simulink model "Australian14gen_inertia"  (R2017b)
settings: Solver=ode23tb  StartTime=0.0  StopTime=50  FixedStep=1e-3  RelTol=1e-3  AbsTol=1e-3  EnableMultiTasking=on
PreLoadFcn:
  | dataaustralian14gen
values from neighbouring files (symbols this model uses):
  alpha = -sys.follin.opt.alpha*1e8    [main_following.m]    (also in optimgains.mat = [-2447350365.29 -12566370614.4 -12566370614.4 -11730281347.7)
  bus_v = [ 101	15 ... (first row only)    [dataaustralian14gen.m]
  comp = [ 1	211	0	0 ... (first row only)    [dataaustralian14gen.m]
  dist = sys.follin.dist    [main_following.m]    (also in main_forming.m = sys.formin.dist)
  Exc = [ 101	0	 200	0.1	    13.25  2.5	 0	0       0       0       0       0 ... (first row only)    [dataaustralian14gen.m]
  FH = 13    [dataaustralian14gen.m]
  FI = 1    [dataaustralian14gen.m]
  FL = .1    (= 0.1)    [dataaustralian14gen.m]
  G_data = [ 101	333.3	15	3.6	0.14	1.1	0.65	0.25	8.5     0.25	0.05	0       0       0.25	0.2 	0 ... (first row only)    [dataaustralian14gen.m]
  KH = 120    [dataaustralian14gen.m]
  KI = 10    [dataaustralian14gen.m]
  KL = 10    [dataaustralian14gen.m]
  Kvsc = [-4.89904313526 -21.043852985 -7.4754770322 -20.8245159401 -7.65455531538 -20.65157337 -7.20128124012 -20.8334958357 -6.74777960012 -20.6206111903 -7.78863485578 -20.7555924998 ... (30 elements, 2x15)]    [optimgains.mat]
  line = [ 102	217	0.0084	0.0667	0.817	330	1 ... (first row only)    [dataaustralian14gen.m]
  load_mag = load_case4    [dataaustralian14gen.m]
  p = p_case4    [dataaustralian14gen.m]
  Pinit = zeros(15,1)    [dataaustralian14gen.m]
  PLL_Ki = 2/500    (= 0.004)    [dataaustralian14gen.m]
  PLL_Kp = 2/500    (= 0.004)    [dataaustralian14gen.m]
  PSSMODEL = 1    [dataaustralian14gen.m]
  trans = [ 1	101	102	15	330	333.3	12	12 ... (first row only)    [dataaustralian14gen.m]
undefined symbols (not defined in the file or in its folder): D1, Delta, sys, thetavsc0, Vbase
libraries: powerlib x388, Library x60, powerlib_meascontrol x15, sps_avr x10, powerlib_extras x4
(part 5 of 5)

== system Australian14gen_inertia/VI504_form ==
  Complex to Magnitude-Angle : ComplexToMagnitudeAngle
  Complex to Magnitude-Angle1 : ComplexToMagnitudeAngle
  Demux : Demux  Outputs=[3 3]
  Filter504 : Library/Filter  r=r_fil  l=l_fil  c=c_fil
  Gain : Gain  Gain=[1 0 0]  Multiplication=Matrix(K*u) (u vector)
  Gain1 : Gain  Gain=[1 0 0]  Multiplication=Matrix(K*u) (u vector)
  INV504 : Library/INV  fn=50  Ub=Vbase(14)  Pref=Pinit(14)  ang=thetavsc0(14)  K2=Kvsc(1,14)  K1=Kvsc(2,14)
  Load Flow Bus17 : powerlib/Measurements/Load Flow Bus  Commented=on  LConnTagsString=a  Phases=single  Connectors=on one side  ID=B504_vsw  Vbase=20e3  Vref=1  Vangle=0  VLF=1  VLFb=1  VLFc=1  angleLF=-12.45  angleLFb=0  angleLFc=0
      settings: AttributesFormatString=%<ID>\n%<Vbase>V\n%<VLF>pu\n%<angleLF>deg.  SourceProductName=Simscape Power Systems
  Mux : Mux  Inputs=2
  Mux1 : Mux  Inputs=2
  Mux21 : Mux  Inputs=3
  Scope : Scope
  Scope1 : Scope  NumInputPorts=2
  Sum : Sum  Inputs=|+-
  fake_VSC_504 : powerlib/Electrical Sources/Three-Phase Source  Commented=on  InternalConnection=Yg  VoltagePhases=off  Voltage=(20000)*1  PhaseAngle=-12.4459  Voltage_phases=[25e3 25e3 25e3]/sqrt(3)  PhaseAngles_phases=[0 -120 +120]  Frequency=50  NonIdealSource=off  SpecifyImpedance=off  Resistance=0  Inductance=0  ShortCircuitLevel=100e6  BaseVoltage=20e3  XRratio=7  BusType=PV  Pref=0  Qref=0  Prefabc=[10e3, 10e3, 10e3]  Qrefabc=[0, 0, 0]  Qmin=-inf  Qmax=inf
  u504 : Constant  Value=0
  A : PMIOPort  Port=1  Side=Left
  B : PMIOPort  Port=2  Side=Left
  C : PMIOPort  Port=3  Side=Left
  tag scope: P504=global, Q504=global, w504=global
  wires:
  INV504/1 -> [P504]
  u504/1 -> INV504/1
  INV504/2 -> Mux21/1
  INV504/3 -> Mux21/2
  Filter504/1 -> INV504/2
  Mux21/1 -> [w504]
  Filter504/2 -> [Q504]
  INV504/4 -> Mux21/3
  Mux/1 -> Scope1/1
  Sum/1 -> Scope/1
  Complex to Magnitude-Angle1/2 -> Mux1/2
  Gain/1 -> Complex to Magnitude-Angle/1
  Complex to Magnitude-Angle/1 -> Mux/1
  Demux/2 -> Gain1/1, Sum/2
  Demux/1 -> Gain/1, Sum/1
  Complex to Magnitude-Angle/2 -> Mux1/1
  Gain1/1 -> Complex to Magnitude-Angle1/1
  Mux1/1 -> Scope1/2
  Complex to Magnitude-Angle1/1 -> Mux/2
  Filter504/3 -> Demux/1
  connections:
  INV504/LConn3 -- fake_VSC_504/RConn3 -- Filter504/LConn3
  Load Flow Bus17/LConn1 -- fake_VSC_504/RConn1 -- INV504/LConn1 -- Filter504/LConn1
  INV504/LConn2 -- fake_VSC_504/RConn2 -- Filter504/LConn2
  C/RConn1 -- Filter504/RConn3
  B/RConn1 -- Filter504/RConn2
  A/RConn1 -- Filter504/RConn1

== system Australian14gen_inertia/VI508 ==
  Constant : Constant  Value=0
  Gain : Gain  Gain=-1
  Gain1 : Gain  Gain=[0 1]  Multiplication=Matrix(K*u) (u vector)
  Mux : Mux  Inputs=2
  Mux1 : Mux  Inputs=3
  PLL : Library/PLL  Kp=PLL_Kp  Ki=PLL_Ki  tau=PLL_tau  theta0=108.332  omega0=0
  "Power (3ph, Phasor)" : powerlib_meascontrol/Measurements/Power (3ph, Phasor)
      settings: SourceProductName=Simscape Power Systems  SourceProductBaseCode=PS
  Three-Phase V-I Measurement : powerlib/Measurements/Three-Phase V-I Measurement  VoltageMeasurement=phase-to-ground  SetLabelV=off  LabelV=Vabc  Vpu=off  VpuLL=off  CurrentMeasurement=yes  SetLabelI=off  LabelI=Iabc  Ipu=off  Pbase=100e6  Vbase=500e3  OutputType=Complex  PhasorSimulation=on  PSBequivalent=0
  dP102_vi : Library/dP102_vi  d=alpha(15)  m=alpha(30)
  virtin : powerlib/Elements/Three-Phase Dynamic Load  NominalVoltage=[ 15e3 50 ]  ActiveReactivePowers=[0 0]  PositiveSequence=[1.00927 -14.4633]  ExternalControl=on  NpNq="[0  0]"  TimeConstants="[0  0  0  0]"  MinimumVoltage=0.01  Tfilter=1e-1  LoadFlowParameters=[4 50000000 0 0 25000000]
      settings: SourceProductName=Simscape Power Systems  SourceProductBaseCode=PS
  A : PMIOPort  Port=1  Side=Right
  B : PMIOPort  Port=2  Side=Right
  C : PMIOPort  Port=3  Side=Right
  tag scope: P508=global, Q508=global, w508=global
  wires:
  Mux/1 -> Gain/1
  Gain/1 -> virtin/1
  Constant/1 -> Mux/2
  dP102_vi/1 -> Mux/1
  [Vabc_B508_vi] -> PLL/1
  PLL/1 -> Mux1/1, dP102_vi/1
  Mux1/1 -> [w508]
  PLL/2 -> Mux1/2, dP102_vi/2
  "Power (3ph, Phasor)"/1 -> [P508]
  Three-Phase V-I Measurement/1 -> "Power (3ph, Phasor)"/1
  "Power (3ph, Phasor)"/2 -> [Q508]
  Three-Phase V-I Measurement/2 -> "Power (3ph, Phasor)"/2
  PLL/3 -> Gain1/1
  Gain1/1 -> Mux1/3
  connections:
  virtin/LConn1 -- Three-Phase V-I Measurement/LConn1
  C/RConn1 -- Three-Phase V-I Measurement/RConn3
  virtin/LConn3 -- Three-Phase V-I Measurement/LConn3
  B/RConn1 -- Three-Phase V-I Measurement/RConn2
  virtin/LConn2 -- Three-Phase V-I Measurement/LConn2
  A/RConn1 -- Three-Phase V-I Measurement/RConn1

== system Australian14gen_inertia/VI508_form ==
  Complex to Magnitude-Angle : ComplexToMagnitudeAngle
  Complex to Magnitude-Angle1 : ComplexToMagnitudeAngle
  Demux : Demux  Outputs=[3 3]
  Filter508 : Library/Filter  r=r_fil  l=l_fil  c=c_fil
  Gain : Gain  Gain=[1 0 0]  Multiplication=Matrix(K*u) (u vector)
  Gain1 : Gain  Gain=[1 0 0]  Multiplication=Matrix(K*u) (u vector)
  INV508 : Library/INV  fn=50  Ub=Vbase(15)  Pref=Pinit(15)  ang=thetavsc0(15)  K2=Kvsc(1,15)  K1=Kvsc(2,15)
  Load Flow Bus19 : powerlib/Measurements/Load Flow Bus  Commented=on  LConnTagsString=a  Phases=single  Connectors=on one side  ID=B508_vsw  Vbase=15e3  Vref=1  Vangle=0  VLF=1  VLFb=1  VLFc=1  angleLF=-14.76  angleLFb=0  angleLFc=0
      settings: AttributesFormatString=%<ID>\n%<Vbase>V\n%<VLF>pu\n%<angleLF>deg.  SourceProductName=Simscape Power Systems
  Mux : Mux  Inputs=2
  Mux1 : Mux  Inputs=2
  Mux20 : Mux  Inputs=3
  Scope : Scope
  Scope1 : Scope  NumInputPorts=2
  Sum : Sum  Inputs=|+-
  fake_VSC_508 : powerlib/Electrical Sources/Three-Phase Source  Commented=on  InternalConnection=Yg  VoltagePhases=off  Voltage=(15000)*1  PhaseAngle=-14.7643  Voltage_phases=[25e3 25e3 25e3]/sqrt(3)  PhaseAngles_phases=[0 -120 +120]  Frequency=50  NonIdealSource=off  SpecifyImpedance=off  Resistance=0  Inductance=0  ShortCircuitLevel=100e6  BaseVoltage=20e3  XRratio=7  BusType=PV  Pref=0  Qref=0  Prefabc=[10e3, 10e3, 10e3]  Qrefabc=[0, 0, 0]  Qmin=-inf  Qmax=inf
  u508 : Constant  Value=0
  A : PMIOPort  Port=1  Side=Left
  B : PMIOPort  Port=2  Side=Left
  C : PMIOPort  Port=3  Side=Left
  tag scope: P508=global, Q508=global, w508=global
  wires:
  Filter508/1 -> INV508/2
  u508/1 -> INV508/1
  INV508/3 -> Mux20/2
  INV508/2 -> Mux20/1
  Filter508/2 -> [Q508]
  INV508/1 -> [P508]
  Mux20/1 -> [w508]
  INV508/4 -> Mux20/3
  Mux/1 -> Scope1/1
  Sum/1 -> Scope/1
  Complex to Magnitude-Angle1/2 -> Mux1/2
  Gain/1 -> Complex to Magnitude-Angle/1
  Complex to Magnitude-Angle/1 -> Mux/1
  Demux/2 -> Gain1/1, Sum/2
  Filter508/3 -> Demux/1
  Demux/1 -> Gain/1, Sum/1
  Complex to Magnitude-Angle/2 -> Mux1/1
  Gain1/1 -> Complex to Magnitude-Angle1/1
  Mux1/1 -> Scope1/2
  Complex to Magnitude-Angle1/1 -> Mux/2
  connections:
  INV508/LConn1 -- fake_VSC_508/RConn1 -- Filter508/LConn1
  INV508/LConn3 -- Load Flow Bus19/LConn1 -- Filter508/LConn3 -- fake_VSC_508/RConn3
  INV508/LConn2 -- fake_VSC_508/RConn2 -- Filter508/LConn2
  A/RConn1 -- Filter508/RConn1
  B/RConn1 -- Filter508/RConn2
  C/RConn1 -- Filter508/RConn3
